simulink model "STOICAL_example_1_Step02b_ActivateParameters"  (R2014b)
settings: Solver=ode4  StartTime=0.0  StopTime=1  FixedStep=50E-6  RelTol=1e-3
model workspace (MAT data in the model file):
  STOVICAL.SignalSaveOptions.ReturnWorkspaceOutputs = 'on'
  STOVICAL.SignalSaveOptions.ReturnWorkspaceOutputsName = 'simout_obj'
  STOVICAL.SignalSaveOptions.SignalLogging = 'on'
  STOVICAL.SignalSaveOptions.SignalLoggingSaveFormat = 'Dataset'
  STOVICAL.SignalSaveOptions.SignalLoggingName = 'STOVICAL_LoggedSignals'
  STOVICAL.ParameterDefinition.BlkNameFull{1} = 'Step amplitude
    | #PARAM#Amplitude'
  STOVICAL.ParameterDefinition.BlkNameFull{2} = 'Static System
    | modelled
    | by gain block
    | #PARAM#SystemGain'
  STOVICAL.ParameterDefinition.BlkNameShort{1} = 'Step amplitude
    | '
  STOVICAL.ParameterDefinition.BlkNameShort{2} = 'Static System
    | modelled
    | by gain block
    | '
  STOVICAL.ParameterDefinition.BlkHandle = [1972.00012207; 1979.00012207]
  STOVICAL.ParameterDefinition.ParamName = {'Amplitude'; 'SystemGain'}
  STOVICAL.ParameterDefinition.BlkPath{1} = 'STOICAL_example_1_Step02b_ActivateParameters/#UNIT#Stimulus/Step amplitude
    | #PARAM#Amplitude'
  STOVICAL.ParameterDefinition.BlkPath{2} = 'STOICAL_example_1_Step02b_ActivateParameters/#UNIT#System/Static System
    | modelled
    | by gain block
    | #PARAM#SystemGain'
  STOVICAL.ParameterDefinition.BlkType = {'Constant'; 'Gain'}
  STOVICAL.ParameterDefinition.BlkMaskType = {''; ''}
  STOVICAL.ParameterDefinition.ParentalBlockPath = {'STOICAL_example_1_Step02b_ActivateParameters/#UNIT#Stimulus'; 'STOICAL_example_1_Step02b_ActivateParameters/#UNIT#System'}
  STOVICAL.ParameterDefinition.ParentalBlockHandle = [1969.00012207; 1977.00036621]
  STOVICAL.ParameterDefinition.Belongs2SubsystemHdl = [1969.00012207; 1977.00036621]
  STOVICAL.ParameterDefinition.NrParams = 2
  STOVICAL.ParameterDefinition.BlkField2Set = {'Value'; 'Gain'}
  STOVICAL.ParameterDefinition.BlkFieldSyntax = {'#'; '#'}
  STOVICAL.ParameterDefinition.ParamVariable = {'param_ec6e274da2c23e664dfdc874ac252818'; 'param_afc1e04cc1c158b687408e5b6ea19d06'}
  STOVICAL.ParameterDefinition.LabelPath = {'#Stimulus#Amplitude'; '#System#SystemGain'}
  STOVICAL.ParameterDefinition.ParamDefaultValue = {'2'; '5'}
undefined symbols (not defined in the file): param_afc1e04cc1c158b687408e5b6ea19d06, param_ec6e274da2c23e664dfdc874ac252818
settings Model: Creator=Wippenbeck  LastModifiedBy=Wippenbeck
settings DataIOCC: ReturnWorkspaceOutputs=on  SignalLoggingName=STOVICAL_LoggedSignals  ReturnWorkspaceOutputsName=simout_obj

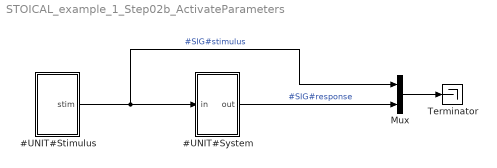
== system STOICAL_example_1_Step02b_ActivateParameters ==
  #UNIT#Stimulus : Subsystem
  #UNIT#System : Subsystem
  Mux : Mux  Inputs=2
  Terminator : Terminator
  wires:
  Mux/1 -> Terminator/1
  #UNIT#Stimulus/1(stim) -> #UNIT#System/1(in), Mux/1  "#SIG#stimulus"
  #UNIT#System/1(out) -> Mux/2  "#SIG#response"

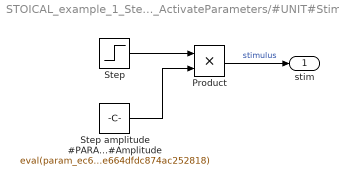
== system STOICAL_example_1_Step02b_ActivateParameters/#UNIT#Stimulus ==
  Product : Product
  Step : Step  Time=0.1  SampleTime=0
  Step amplitude #PARAM#Amplitude : Constant  Value=eval(param_ec6e274da2c23e664dfdc874ac252818)
  stim : Outport
  wires:
  Step amplitude #PARAM#Amplitude/1 -> Product/2
  Product/1 -> stim/1  "stimulus"
  Step/1 -> Product/1

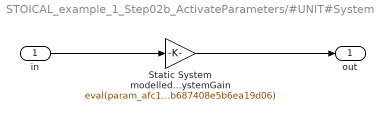
== system STOICAL_example_1_Step02b_ActivateParameters/#UNIT#System ==
  in : Inport
  Static System modelled by gain block #PARAM#SystemGain : Gain  Gain=eval(param_afc1e04cc1c158b687408e5b6ea19d06)
  out : Outport
  wires:
  Static System modelled by gain block #PARAM#SystemGain/1 -> out/1
  in/1 -> Static System modelled by gain block #PARAM#SystemGain/1
